simulink model "Schematb"  (R2018a)
settings: Solver=VariableStepAuto  StartTime=0.0  StopTime=10.0  RelTol=1e-3
values from neighbouring files (symbols this model uses):
  czas_skok = 50000    [Skrypt.m]
  dTkz0 = 0    [Skrypt.m]
  dTzew0 = 0    [Skrypt.m]
  L11 = [Cv2*cp*rop*fk, cp*rop*fk*(k0+cp*rop*fk+ks2)]    [Skrypt.m]
  L12 = [ks1*Cv2, ks1*(k0+cp*rop*fk+ks2)+k0*ks2]    [Skrypt.m]
  L21 = [k0*cp*rop*fk+(cp*rop*fk)^2]    [Skrypt.m]
  L22 = [ks2*Cv1, ks2*(cp*rop*fk+ks1+k0)+k0+ks1+cp*rop*fk*ks1]    [Skrypt.m]
  M = [Cv1*Cv2, Cv1*(k0+cp*rop*fk+ks2)+Cv2*(cp*rop*fk+ks1+k0), (cp*rop*fk+ks1+k0)*(cp*rop*fk+ks2+k0)-k0^2-k0*cp*rop*fk]    [Skrypt.m]
  Tw10 = ((k0+cp*rop*fk0+ks2)*(cp*rop*fk0*Tkz0+ks1*Tzew0)+k0*ks2*Tzew0)/((cp*rop*fk0+ks1+k0)*(k0+cp*rop*fk0+ks2)-k0*(k0+cp*rop*fk0))    (= 20)    [Skrypt.m]
  Tw20 = (Tw10*(k0+cp*rop*fk0)+ks2*Tzew0)/(k0+cp*rop*fk0+ks2)    (= 15)    [Skrypt.m]
  Tzew0 = Tzewn + 0    (= -20)    [Skrypt.m]
settings Model: Creator=Mutungamiri  LastModifiedBy=Mutungamiri

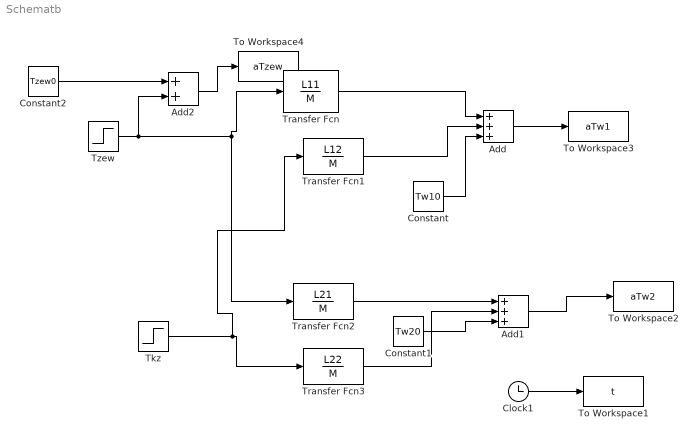
== system Schematb ==
  Add : Sum  Inputs=+++
  Add1 : Sum  Inputs=+++
  Add2 : Sum
  Clock1 : Clock
  Constant : Constant  Value=Tw10
  Constant1 : Constant  Value=Tw20
  Constant2 : Constant  Value=Tzew0
  Tkz : Step  Time=czas_skok  After=dTkz0  SampleTime=0
  To Workspace1 : ToWorkspace  VariableName=t  SampleTime=-1
  To Workspace2 : ToWorkspace  VariableName=aTw2  SampleTime=-1
  To Workspace3 : ToWorkspace  VariableName=aTw1  SampleTime=-1
  To Workspace4 : ToWorkspace  VariableName=aTzew  SampleTime=-1
  Transfer Fcn : TransferFcn  Numerator=L11  Denominator=M
  Transfer Fcn1 : TransferFcn  Numerator=L12  Denominator=M
  Transfer Fcn2 : TransferFcn  Numerator=L21  Denominator=M
  Transfer Fcn3 : TransferFcn  Numerator=L22  Denominator=M
  Tzew : Step  Time=czas_skok  After=dTzew0  SampleTime=0
  wires:
  Add/1 -> To Workspace3/1
  Add1/1 -> To Workspace2/1
  Transfer Fcn2/1 -> Add1/1
  Transfer Fcn3/1 -> Add1/2
  Transfer Fcn/1 -> Add/1
  Transfer Fcn1/1 -> Add/2
  Tzew/1 -> Add2/2, Transfer Fcn/1, Transfer Fcn2/1
  Tkz/1 -> Transfer Fcn1/1, Transfer Fcn3/1
  Constant/1 -> Add/3
  Constant1/1 -> Add1/3
  Clock1/1 -> To Workspace1/1
  Constant2/1 -> Add2/1
  Add2/1 -> To Workspace4/1
